simulink model "PT1_estimation_and_Parameter_Adaption"  (R2018b)
settings: Solver=VariableStepAuto  StartTime=0  StopTime=50  FixedStep=0.1  MaxStep=0.5  RelTol=1e-3  EnableMultiTasking=on
undefined symbols (not defined in the file): idss, Ts, u0, x0, y0
libraries: slident x5, simulink x4, mpclib x2
settings Model: Creator=The MathWorks, Inc.  LastModifiedBy=Trips
settings DataIOCC: ExternalInput=ExtIn  InitialState=[311.267; 8.5695]  SaveFormat=Structure  SaveOutput=off  SignalLogging=off  DSMLogging=off  SaveTime=off  SignalLoggingName=logsOut
settings OptimizationCC: BooleanDataType=off  DefaultParameterBehavior=Inlined  InlineInvariantSignals=on  BufferReuse=off  ExpressionDepthLimit=2147483647  InitFltsAndDblsToZero=on  LifeSpan=inf
settings DebuggingCC: SaveWithParameterizedLinksMsg=none  UnderspecifiedInitializationDetection=Classic  MergeDetectMultiDrivingBlocksExec=none  CheckExecutionContextPreStartOutputMsg=on  CheckExecutionContextRuntimeOutputMsg=on  SignalResolutionControl=TryResolveAllWithWarning  MultiTaskDSMMsg=warning  MultiTaskCondExecSysMsg=none  StateNameClashWarn=warning  LibraryContextMissingDiagnostic=none  SFUnexpectedBacktrackingDiag=warning  SFNoUnconditionalDefaultTransitionDiag=warning  SFExecutionAtInitializationDiag=none  UnderSpecifiedDimensionMsg=warning
settings HardwareCC: ProdBitPerPointer=32  ProdBitPerSizeT=32  ProdBitPerPtrDiffT=32  ProdLargestAtomicFloat=None  ProdIntDivRoundTo=Undefined  ProdEndianess=Unspecified  ProdWordSize=32  ProdHWDeviceType=32-bit Generic  TargetUnknown=on
settings ModelReferenceCC: PropagateSignalLabelsOutOfModel=off
settings SFSimCC: SimUseLocalCustomCode=off
settings RTWCC: RTWUseLocalCustomCode=off
settings CodeAppCC: StateflowObjectComments=on
settings GRTTargetCC: TargetFcnLib=ansi_tfl_tmw.mat  TargetLangStandard=C89/C90 (ANSI)  GeneratePreprocessorConditionals=Disable all  CombineOutputUpdateFcns=off  GRTInterface=on
settings ConfigComp: CovMetricSettings=dw  CovHtmlReporting=on  CovSaveCumulativeToWorkspaceVar=on  CovSaveSingleToWorkspaceVar=on  CovExternalEMLEnable=off  CovSFcnEnable=off

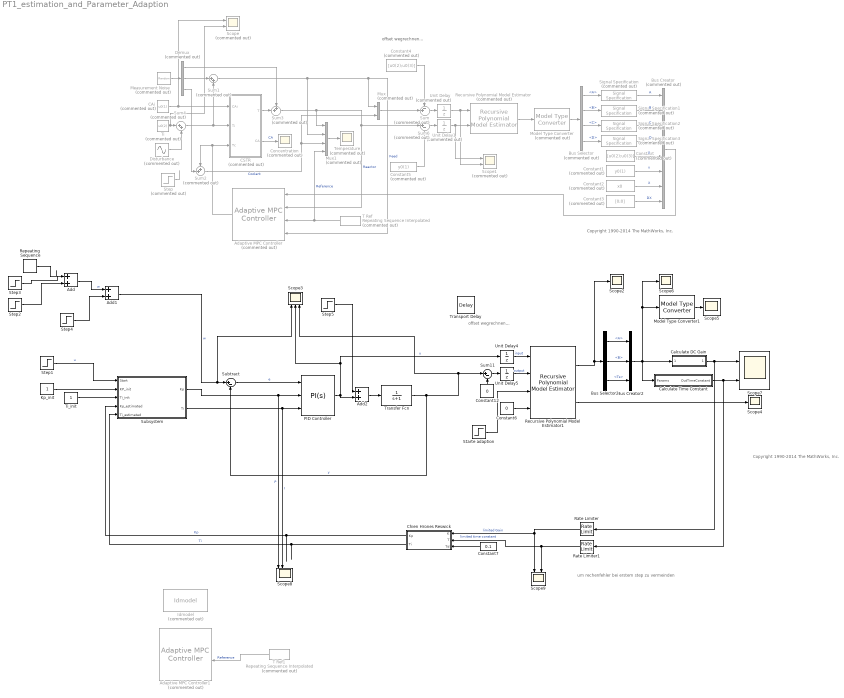
== system PT1_estimation_and_Parameter_Adaption ==
  note: um rechenfehler bei erstem step zu vermeinden
  note: offset wegrechnen...
  note: Copyright 1990-2014 The MathWorks, Inc.
  note: Copyright 1990-2014 The MathWorks, Inc.
  note: offset wegrechnen...
  Adaptive MPC Controller : mpclib/Adaptive MPC Controller  Commented=on  SCDEnableBlockLinearizationSpecification=on  mpcobj=mpcobj  enable_value=0  updateMPCinCallerWorkspace=on  md_inport=on  mv_inport=off  return_cost=off  return_mvseq=off  return_qpstatus=off  return_xseq=off  return_state=off  return_ovseq=off  state_inport=off  isltv_plant=off  umin_inport=off  umax_inport=off  ymin_inport=off  ymax_inport=off  cc_inport=off  ywt_inport=off  uwt_inport=off  duwt_inport=off  rhoeps_inport=off  uref_inport=off  BlockDataType=double  SampleTimeInherited=off  switch_inport=off
      settings: SourceProductName=Model Predictive Control Toolbox
  Adaptive MPC Controller1 : mpclib/Adaptive MPC Controller  Commented=on  SCDEnableBlockLinearizationSpecification=on  mpcobj=mpcPT1  enable_value=0  updateMPCinCallerWorkspace=on  md_inport=on  mv_inport=off  return_cost=off  return_mvseq=off  return_qpstatus=off  return_xseq=off  return_state=off  return_ovseq=off  state_inport=off  isltv_plant=off  umin_inport=off  umax_inport=off  ymin_inport=off  ymax_inport=off  cc_inport=off  ywt_inport=off  uwt_inport=off  duwt_inport=off  rhoeps_inport=off  uref_inport=off  BlockDataType=double  SampleTimeInherited=off  switch_inport=off
      settings: SourceProductName=Model Predictive Control Toolbox
  Add : Sum
  Add1 : Sum
  Add2 : Sum
  Bus Creator : BusCreator  Commented=on  Inputs=8
  Bus Creator2 : BusCreator  Inputs=3
  Bus Selector : BusSelector  Commented=on  OutputSignals=A,B,C,D
  Bus Selector2 : BusSelector  OutputSignals=A,B,Ts
  CAi : Constant  Commented=on  Value=u0(1)
  CSTR : Subsystem  Commented=on
  Calculate DC Gain : Subsystem
  Calculate Time Constant : Subsystem
  Chien Hrones Reswick : Subsystem
  Concentration : Scope  Commented=on
  Constant : Constant  Commented=on  Value=[u0(2);u0(3)]  VectorParams1D=off
  Constant1 : Constant  Commented=on  Value=y0(1)  VectorParams1D=off
  Constant12 : Constant  Value=0
  Constant2 : Constant  Commented=on  Value=x0  VectorParams1D=off
  Constant3 : Constant  Commented=on  Value=[0;0]  VectorParams1D=off
  Constant4 : Constant  Commented=on  Value=[u0(2);u0(3)]
  Constant5 : Constant  Commented=on  Value=y0(1)
  Constant6 : Constant  Value=0
  Constant7 : Constant  Value=0.1
  Demux : Demux  Commented=on  Outputs=3
  Disturbance : Sin  Commented=on  Amplitude=5  Frequency=0.05  SampleTime=0
  Idmodel : slident/Models/Idmodel  Commented=on  sys=idss(-1,1,1,0,'Ts',1)  IC=0  noi=on  seed=[]
      settings: SourceProductName=System Identification Toolbox  SourceProductBaseCode=ID
  Kp_init : Constant
  Measurement Noise : RandomNumber  Commented=on  Mean=[0 0 0]  Variance=0.001*[1 1 1]  Seed=12345  SampleTime=Ts/5
  Model Type Converter : slident/Estimators/Model Type Converter  Commented=on  InputModelType=ARX
      settings: SourceProductName=System Identification Toolbox  SourceProductBaseCode=ID
  Model Type Converter1 : slident/Estimators/Model Type Converter  InputModelType=ARX
      settings: SourceProductName=System Identification Toolbox  SourceProductBaseCode=ID
  Mux : Mux  Commented=on  Inputs=2
  Mux1 : Mux  Commented=on
  PID Controller : simulink/Continuous/PID Controller  Controller=PI  Form=Ideal  TimeDomain=Continuous-time  SampleTime=-1  IntegratorMethod=Forward Euler  FilterMethod=Forward Euler  ControllerParametersSource=external  P=1.04240469046453  I=3.00115000619232  D=0  UseFilter=on  N=100  TunerSelectOption=Transfer Function Based (PID Tuner App)  InitialConditionSource=internal  InitialConditionForIntegrator=0  InitialConditionForFilter=0  DifferentiatorICPrevScaledInput=0  ExternalReset=none  TrackingMode=off  Kt=1  LimitOutput=off  UpperSaturationLimit=inf  LowerSaturationLimit=-inf  LinearizeAsGain=on  AntiWindupMode=none  Kb=1  POutMin=[]  POutMax=[]  IOutMin=[]  IOutMax=[]  DOutMin=[]  DOutMax=[]  NOutMin=[]  NOutMax=[]  SumOutMin=[]  SumOutMax=[]  SaturationOutMin=[]  SaturationOutMax=[]  PParamMin=[]  PParamMax=[]  IParamMin=[]  IParamMax=[]  DParamMin=[]  DParamMax=[]  NParamMin=[]  NParamMax=[]  KbParamMin=[]  KbParamMax=[]  KtParamMin=[]  KtParamMax=[]  KbOutMin=[]  KbOutMax=[]  KtOutMin=[]  KtOutMax=[]  IntegratorOutMin=[]  IntegratorOutMax=[]  FilterOutMin=[]  FilterOutMax=[]  SumI1OutMin=[]  SumI1OutMax=[]  SumI2OutMin=[]  SumI2OutMax=[]  SumI3OutMin=[]  SumI3OutMax=[]  SumI4OutMin=[]  SumI4OutMax=[]  SumDOutMin=[]  SumDOutMax=[]  DifferentiatorOutMin=[]  DifferentiatorOutMax=[]  FilterDiffOutCoefMin=[]  FilterDiffOutCoefMax=[]  ReciprocalOutMin=[]  ReciprocalOutMax=[]  SumDenOutMin=[]  SumDenOutMax=[]  SumNumOutMin=[]  SumNumOutMax=[]  DivideOutMin=[]  DivideOutMax=[]  IntegratorContinuousStateAttributes=''  IntegratorStateMustResolveToSignalObject=off  IntegratorRTWStateStorageClass=Auto  FilterContinuousStateAttributes=''  FilterStateMustResolveToSignalObject=off  FilterRTWStateStorageClass=Auto  ParallelPVariant=Passthrough  IdealPVariant=ExternalParameters  IVariant=ExternalParameters  DVariant=Disabled  IntegratorVariant=Continuous  SatVariant=Disabled  AWVariant=Passthrough  PCopyVariant=Disabled  TRVariant=Disabled  FdbkBlocksVariant=Forward  IdealPFdbkVariant=Disabled  SatFdbkVariant=Disabled  DerivativeFilterVariant=Disabled  NVariant=Disabled  NCopyVariant=Disabled_SignalSpec  FilterICVariant=Disabled  IntegratorICVariant=InternalICs  ExternalResetVariant=Disabled  TRSumVariant=Passthrough  SumFdbkVariant=Disabled  SumVariant=Sum_PI
  Rate Limiter : RateLimiter  SampleTimeMode=inherited
  Rate Limiter1 : RateLimiter  SampleTimeMode=inherited
  Recursive Polynomial Model Estimator : slident/Estimators/Recursive Polynomial Model Estimator  Commented=on  ModelStructure=ARX  InitialEstimateSource=Internal  A0=Aq  B0=Bq  C0=1  D0=1  F0=1  nk=1  P0=1  InitialInputs=0  InitialOutputs=0  History=Infinite  WindowLength=200  EstimationMethod=Kalman Filter  AdaptationParameter=0.01  HasTimeVaryingAdaptationParameter=off  NormalizationBias=eps  OutputError=off  OutputP=off  AddEnablePort=off  InputProcessing=Sample-based  Ts=Ts
      settings: SourceProductName=System Identification Toolbox  SourceProductBaseCode=ID
  Recursive Polynomial Model Estimator1 : slident/Estimators/Recursive Polynomial Model Estimator  ModelStructure=ARX  InitialEstimateSource=None  A0=1  B0=1  C0=1  D0=1  F0=1  nk=0  P0=1  InitialInputs=0  InitialOutputs=0  History=Infinite  WindowLength=10  EstimationMethod=Forgetting Factor  AdaptationParameter=1  HasTimeVaryingAdaptationParameter=off  NormalizationBias=eps  OutputError=on  OutputP=off  AddEnablePort=on  ExternalReset=Rising  InputProcessing=Sample-based  Ts=0.1
      settings: SourceProductName=System Identification Toolbox  SourceProductBaseCode=ID
  Repeating Sequence : simulink/Sources/Repeating Sequence  rep_seq_t=[0 5 8 13]  rep_seq_y=[0 0.6 0.6 0]
  Scope : Scope  Commented=on  NumInputPorts=2
  Scope1 : Scope  Commented=on  NumInputPorts=2
  Scope{2,4..6} (4 alike) : Scope
  Scope3 : Scope  NumInputPorts=3
  Scope7 : Scope  NumInputPorts=2
  Scope8 : Scope  NumInputPorts=4
  Scope9 : Scope  NumInputPorts=2
  Signal Specification : SignalSpecification  Commented=on  Dimensions=[2 2]
  Signal Specification1 : SignalSpecification  Commented=on  Dimensions=[2 2]
  Signal Specification2 : SignalSpecification  Commented=on  Dimensions=[1 2]
  Signal Specification3 : SignalSpecification  Commented=on  Dimensions=[1 2]
  Starte adaption : Step  Time=0  SampleTime=0.1
  Step : Step  Commented=on  Time=75  After=10  SampleTime=0
  Step1 : Step  SampleTime=0
  Step2 : Step  Time=0  After=2.7  SampleTime=0
  Step3 : Step  Time=10  After=-1  SampleTime=0
  Step4 : Step  Time=15  SampleTime=0
  Step5 : Step  Time=25  After=5  SampleTime=0
  Subsystem : Subsystem
  Subtract : Sum  Inputs=|+-
  Sum : Sum  Commented=on  Inputs=-+|
  Sum1 : Sum  Commented=on  Inputs=|++  SampleTime=Ts/5
  Sum11 : Sum  Inputs=|+-
  Sum2 : Sum  Commented=on  Inputs=++|  SampleTime=Ts/5
  Sum3 : Sum  Commented=on  Inputs=++|  SampleTime=Ts/5
  Sum4 : Sum  Commented=on  Inputs=|++  SampleTime=Ts/5
  Sum6 : Sum  Commented=on  Inputs=|+-
  T Ref : simulink/Sources/Repeating Sequence Interpolated  Commented=on  OutValues=[y0(1) y0(1) 373 373]  TimeValues=[0 50 100 150]  LookUpMeth=Interpolation-Use End Values  tsamp=Ts  OutMin=[]  OutMax=[]  OutDataTypeStr=double  OutputDataTypeScalingMode=double  OutDataType=fixdt(0,8)  OutScaling=2^-10
  T Ref1 : simulink/Sources/Repeating Sequence Interpolated  Commented=on  OutValues=[y0(1) y0(1) 373 373]  TimeValues=[0 50 100 150]  LookUpMeth=Interpolation-Use End Values  tsamp=Ts  OutMin=[]  OutMax=[]  OutDataTypeStr=double  OutputDataTypeScalingMode=double  OutDataType=fixdt(0,8)  OutScaling=2^-10
  Temperature : Scope  Commented=on
  Ti : Constant  Commented=on  Value=u0(2)
  Ti_init : Constant
  Transfer Fcn : TransferFcn  Denominator=[1 1]
  Transport Delay : TransportDelay  DelayTime=0.2
  Unit Delay : UnitDelay  Commented=on  InitialCondition=[0;0]  SampleTime=Ts
  Unit Delay1 : UnitDelay  Commented=on  SampleTime=Ts
  Unit Delay4 : UnitDelay  InitialCondition=[0]  SampleTime=0.1
  Unit Delay5 : UnitDelay  SampleTime=0.1
  wires:
  Mux1/1 -> Temperature/1
  Sum1/1 -> Adaptive MPC Controller/4, Mux/1, Mux1/2  "Feed"
  Bus Creator/1 -> Adaptive MPC Controller/1
  Sum2/1 -> Mux/2, Mux1/3  "Coolant"
  Sum3/1 -> Adaptive MPC Controller/2, Sum6/1, Mux1/1  "Reactor"
  CSTR/2(CA) -> Concentration/1  "CA"
  CSTR/1(T) -> Sum3/2
  Ti/1 -> Scope/2, Sum4/1
  Sum4/1 -> Sum1/2, CSTR/2(Ti)
  T Ref/1 -> Adaptive MPC Controller/3, Mux1/4  "Reference"
  Disturbance/1 -> Sum4/2
  Demux/2 -> Sum1/1
  Demux/1 -> Sum3/1
  Demux/3 -> Sum2/2
  Measurement Noise/1 -> Demux/1
  Unit Delay1/1 -> Scope1/1, Recursive Polynomial Model Estimator/2
  Model Type Converter/1 -> Bus Selector/1
  Recursive Polynomial Model Estimator/1 -> Model Type Converter/1
  Constant1/1 -> Bus Creator/6  "Y"
  Constant/1 -> Bus Creator/5  "U"
  Bus Selector/1 -> Signal Specification/1  "<A>"
  Signal Specification/1 -> Bus Creator/1  "A"
  Bus Selector/2 -> Signal Specification1/1  "<B>"
  Bus Selector/3 -> Signal Specification2/1  "<C>"
  Bus Selector/4 -> Signal Specification3/1  "<D>"
  Signal Specification1/1 -> Bus Creator/2  "B"
  Signal Specification2/1 -> Bus Creator/3  "C"
  Signal Specification3/1 -> Bus Creator/4  "D"
  Constant2/1 -> Bus Creator/7  "X"
  Constant3/1 -> Bus Creator/8  "DX"
  Adaptive MPC Controller/1 -> Sum2/1, CSTR/3(Tc)
  Sum6/1 -> Unit Delay1/1
  Sum/1 -> Unit Delay/1
  Mux/1 -> Sum/2
  Constant4/1 -> Sum/1
  Unit Delay/1 -> Scope1/2, Recursive Polynomial Model Estimator/1
  Constant5/1 -> Sum6/2
  CAi/1 -> Scope/1, CSTR/1(CAi)
  Step/1 -> ?
  Unit Delay4/1 -> Recursive Polynomial Model Estimator1/1  "input"
  Sum11/1 -> Unit Delay5/1
  T Ref1/1 -> Adaptive MPC Controller1/3  "Reference"
  Unit Delay5/1 -> Recursive Polynomial Model Estimator1/2  "output"
  Constant12/1 -> Sum11/2
  Recursive Polynomial Model Estimator1/2 -> Scope4/1
  Model Type Converter1/1 -> Scope5/1
  Recursive Polynomial Model Estimator1/1 -> Scope2/1, Bus Selector2/1
  Bus Selector2/3 -> Bus Creator2/3  "<Ts>"
  Bus Selector2/2 -> Bus Creator2/2  "<B>"
  Bus Selector2/1 -> Bus Creator2/1  "<A>"
  Bus Creator2/1 -> Calculate Time Constant/1(Params), Calculate DC Gain/1(Params), Scope6/1, Model Type Converter1/1
  Starte adaption/1 -> Recursive Polynomial Model Estimator1/3
  Step2/1 -> Add/2
  Transfer Fcn/1 -> Subtract/2, Scope3/3, Sum11/1  "y"
  Repeating Sequence/1 -> ?
  Constant6/1 -> Recursive Polynomial Model Estimator1/4
  Add1/1 -> Scope3/1, Subtract/1  "w"
  Step1/1 -> Subsystem/1(Start)  "u"
  Chien Hrones Reswick/1(Kp) -> Subsystem/4(Kp_estimated)  "Kp"
  Chien Hrones Reswick/2(Ti) -> Subsystem/5(Ti_estimated)  "Ti"
  Constant7/1 -> Chien Hrones Reswick/3(Td)
  Kp_init/1 -> Subsystem/2(KP_init)
  Subsystem/1(Kp) -> Scope8/1, PID Controller/2  "P"
  Subsystem/2(Ti) -> PID Controller/3, Scope8/2  "I"
  Ti_init/1 -> Subsystem/3(Ti_init)
  Subtract/1 -> PID Controller/1  "e"
  Step3/1 -> Add/1
  Add/1 -> Add1/1  "w"
  Step4/1 -> Add1/2
  PID Controller/1 -> Add2/2, Unit Delay4/1, Scope3/2  "u"
  Calculate DC Gain/1(DCGain) -> Rate Limiter/1, Scope7/1
  Calculate Time Constant/1("OutTimeConstant ") -> Rate Limiter1/1, Scope7/2
  Rate Limiter1/1 -> Chien Hrones Reswick/2(T), Scope9/2  "limited time constant"
  Rate Limiter/1 -> Scope9/1, Chien Hrones Reswick/1(K)  "limited Gain"
  Add2/1 -> Transfer Fcn/1
  Step5/1 -> Add2/1

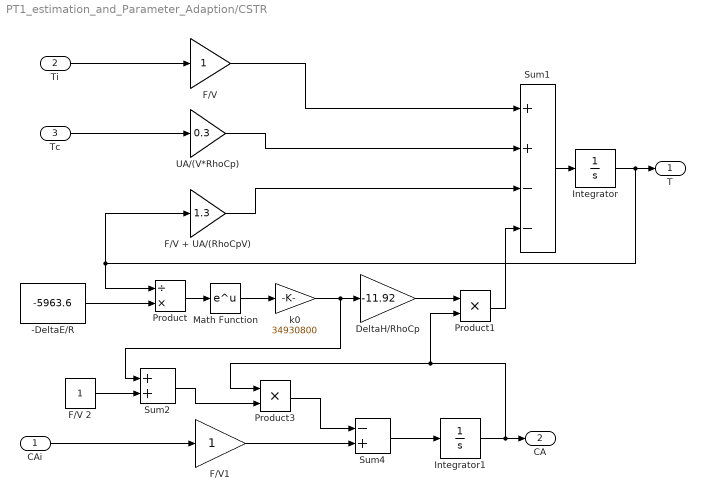
== system PT1_estimation_and_Parameter_Adaption/CSTR ==
  CAi : Inport
  Ti : Inport  Port=2
  Tc : Inport  Port=3
  -DeltaE/R : Constant  Value=-5963.6
  DeltaH/RhoCp : Gain  Gain=-11.92  SaturateOnIntegerOverflow=on  OutDataTypeStr=Inherit: Same as input  ParamDataTypeStr=Inherit: Same as input
  F/V : Gain  SaturateOnIntegerOverflow=on  OutDataTypeStr=Inherit: Same as input  ParamDataTypeStr=Inherit: Same as input
  F/V + UA/(RhoCpV) : Gain  Gain=1.3  SaturateOnIntegerOverflow=on  OutDataTypeStr=Inherit: Same as input  ParamDataTypeStr=Inherit: Same as input
  F/V 2 : Constant
  F/V1 : Gain  SaturateOnIntegerOverflow=on  OutDataTypeStr=Inherit: Same as input  ParamDataTypeStr=Inherit: Same as input
  Integrator : Integrator  InitialCondition=311.2639  LimitOutput=on  LowerSaturationLimit=0
  Integrator1 : Integrator  InitialCondition=8.5698  LimitOutput=on  LowerSaturationLimit=0
  Math Function : Math  SaturateOnIntegerOverflow=on
  Product : Product  Inputs=/*  SaturateOnIntegerOverflow=on  RndMeth=Zero  InputSameDT=on  OutDataTypeStr=Inherit: Same as first input
  Product1 : Product  SaturateOnIntegerOverflow=on  RndMeth=Zero  InputSameDT=on  OutDataTypeStr=Inherit: Same as first input
  Product3 : Product  SaturateOnIntegerOverflow=on  RndMeth=Zero  InputSameDT=on  OutDataTypeStr=Inherit: Same as first input
  Sum1 : Sum  Inputs=++--  SaturateOnIntegerOverflow=on  InputSameDT=on  OutDataTypeStr=Inherit: Same as first input
  Sum2 : Sum  SaturateOnIntegerOverflow=on  InputSameDT=on  OutDataTypeStr=Inherit: Same as first input
  Sum4 : Sum  Inputs=-+  SaturateOnIntegerOverflow=on  InputSameDT=on  OutDataTypeStr=Inherit: Same as first input
  UA/(V*RhoCp) : Gain  Gain=0.3  SaturateOnIntegerOverflow=on  OutDataTypeStr=Inherit: Same as input  ParamDataTypeStr=Inherit: Same as input
  k0 : Gain  Gain=34930800  SaturateOnIntegerOverflow=on  OutDataTypeStr=Inherit: Same as input  ParamDataTypeStr=Inherit: Same as input
  T : Outport
  CA : Outport  Port=2
  wires:
  Sum2/1 -> Product3/2
  Tc/1 -> UA/(V*RhoCp)/1
  CAi/1 -> F/V1/1
  Ti/1 -> F/V/1
  F/V1/1 -> Sum4/2
  F/V 2/1 -> Sum2/2
  Integrator1/1 -> CA/1, Product3/1, Product1/2
  Sum4/1 -> Integrator1/1
  Product3/1 -> Sum4/1
  -DeltaE/R/1 -> Product/2
  k0/1 -> Sum2/1, DeltaH/RhoCp/1
  Product1/1 -> Sum1/4
  DeltaH/RhoCp/1 -> Product1/1
  Math Function/1 -> k0/1
  Product/1 -> Math Function/1
  F/V + UA/(RhoCpV)/1 -> Sum1/3
  UA/(V*RhoCp)/1 -> Sum1/2
  Integrator/1 -> T/1, F/V + UA/(RhoCpV)/1, Product/1
  Sum1/1 -> Integrator/1
  F/V/1 -> Sum1/1

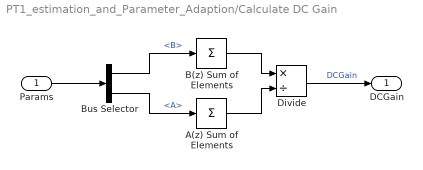
== system PT1_estimation_and_Parameter_Adaption/Calculate DC Gain ==
  Params : Inport
  A(z) Sum of Elements : Sum  Inputs=+
  B(z) Sum of Elements : Sum  Inputs=+
  Bus Selector : BusSelector  OutputSignals=B,A
  Divide : Product  Inputs=*/
  DCGain : Outport
  wires:
  A(z) Sum of Elements/1 -> Divide/2
  B(z) Sum of Elements/1 -> Divide/1
  Params/1 -> Bus Selector/1
  Bus Selector/1 -> B(z) Sum of Elements/1  "<B>"
  Bus Selector/2 -> A(z) Sum of Elements/1  "<A>"
  Divide/1 -> DCGain/1  "DCGain"

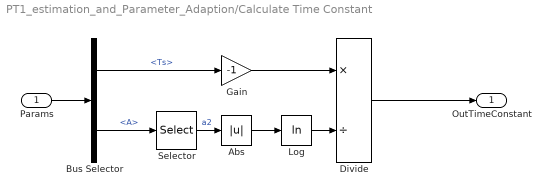
== system PT1_estimation_and_Parameter_Adaption/Calculate Time Constant ==
  Params : Inport
  Abs : Abs
  Bus Selector : BusSelector  OutputSignals=Ts,A
  Divide : Product  Inputs=*/
  Gain : Gain  Gain=-1
  Log : Math  Operator=log  SaturateOnIntegerOverflow=on
  Selector : Selector  InputPortWidth=2  IndexOptions=Starting index (dialog)  Indices=[2]  OutputSizes=1
  "OutTimeConstant " : Outport
  wires:
  Params/1 -> Bus Selector/1
  Bus Selector/1 -> Gain/1  "<Ts>"
  Bus Selector/2 -> Selector/1  "<A>"
  Selector/1 -> Abs/1  "a2"
  Gain/1 -> Divide/1
  Log/1 -> Divide/2
  Divide/1 -> "OutTimeConstant "/1
  Abs/1 -> Log/1

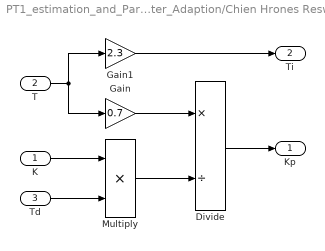
== system PT1_estimation_and_Parameter_Adaption/Chien Hrones Reswick ==
  K : Inport
  T : Inport  Port=2
  Td : Inport  Port=3
  Divide : Product  Inputs=*/
  Gain : Gain  Gain=0.7
  Gain1 : Gain  Gain=2.3
  Multiply : Product
  Kp : Outport
  Ti : Outport  Port=2
  wires:
  T/1 -> Gain/1, Gain1/1
  Gain/1 -> Divide/1
  Td/1 -> Multiply/2
  Multiply/1 -> Divide/2
  Divide/1 -> Kp/1
  K/1 -> Multiply/1
  Gain1/1 -> Ti/1

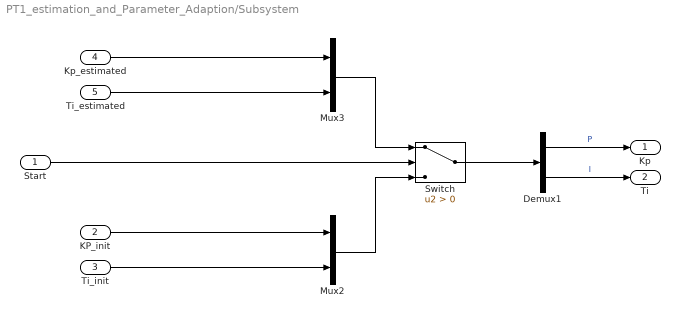
== system PT1_estimation_and_Parameter_Adaption/Subsystem ==
  Start : Inport
  KP_init : Inport  Port=2
  Ti_init : Inport  Port=3
  Kp_estimated : Inport  Port=4
  Ti_estimated : Inport  Port=5
  Demux1 : Demux  Outputs=2
  Mux2 : Mux  Inputs=2
  Mux3 : Mux  Inputs=2
  Switch : Switch  Criteria=u2 > Threshold
  Kp : Outport
  Ti : Outport  Port=2
  wires:
  Mux3/1 -> Switch/1
  Mux2/1 -> Switch/3
  Start/1 -> Switch/2
  Switch/1 -> Demux1/1
  KP_init/1 -> Mux2/1
  Ti_init/1 -> Mux2/2
  Kp_estimated/1 -> Mux3/1
  Ti_estimated/1 -> Mux3/2
  Demux1/1 -> Kp/1  "P"
  Demux1/2 -> Ti/1  "I"
